simulink model "sampleModel7424_pp_1_1"  (R2018a)
settings: Solver=VariableStepAuto  StartTime=0.0  StopTime=10.0  RelTol=1e-3
undefined symbols (not defined in the file): DiscIntNeverNeededParam
libraries: simulink x211
(part 6 of 7)

== matlab function sampleModel7424_pp_1_1/cfblk142/cfblk19/emi_11 ==
  data: o input; e input
function  fcn(o, e)
o_inv = o^-1;
e_inv = e^-1;

emsg = 'sampleModel7424_pp_1_1/cfblk142/cfblk19/emi_11';
 
if(o == e)
    assert(o_inv == e_inv, [emsg ' ; o_inv~=e_inv']);
    return;
end
 
if(o_inv > 0)
    assert(e_inv < 0, [emsg ' ; e_inv>=0']);
else
    assert(e_inv > 0, [emsg ' ; e_inv<=0']);
end

== matlab function sampleModel7424_pp_1_1/cfblk134/emi_13 ==
  data: o input; e input
function  fcn(o, e)
o_inv = o^-1;
e_inv = e^-1;

emsg = 'sampleModel7424_pp_1_1/cfblk134/emi_13';
 
if(o == e)
    assert(o_inv == e_inv, [emsg ' ; o_inv~=e_inv']);
    return;
end
 
if(o_inv > 0)
    assert(e_inv < 0, [emsg ' ; e_inv>=0']);
else
    assert(e_inv > 0, [emsg ' ; e_inv<=0']);
end

== matlab function sampleModel7424_pp_1_1/cfblk148/emi_15 ==
  data: o input; e input
function  fcn(o, e)
o_inv = o^-1;
e_inv = e^-1;

emsg = 'sampleModel7424_pp_1_1/cfblk148/emi_15';
 
if(o == e)
    assert(o_inv == e_inv, [emsg ' ; o_inv~=e_inv']);
    return;
end
 
if(o_inv > 0)
    assert(e_inv < 0, [emsg ' ; e_inv>=0']);
else
    assert(e_inv > 0, [emsg ' ; e_inv<=0']);
end

== matlab function sampleModel7424_pp_1_1/cfblk127/emi_17 ==
  data: o input; e input
function  fcn(o, e)
o_inv = o^-1;
e_inv = e^-1;

emsg = 'sampleModel7424_pp_1_1/cfblk127/emi_17';
 
if(o == e)
    assert(o_inv == e_inv, [emsg ' ; o_inv~=e_inv']);
    return;
end
 
if(o_inv > 0)
    assert(e_inv < 0, [emsg ' ; e_inv>=0']);
else
    assert(e_inv > 0, [emsg ' ; e_inv<=0']);
end

== matlab function sampleModel7424_pp_1_1/cfblk127/cfblk19/emi_19 ==
  data: o input; e input
function  fcn(o, e)
o_inv = o^-1;
e_inv = e^-1;

emsg = 'sampleModel7424_pp_1_1/cfblk127/cfblk19/emi_19';
 
if(o == e)
    assert(o_inv == e_inv, [emsg ' ; o_inv~=e_inv']);
    return;
end
 
if(o_inv > 0)
    assert(e_inv < 0, [emsg ' ; e_inv>=0']);
else
    assert(e_inv > 0, [emsg ' ; e_inv<=0']);
end

== matlab function sampleModel7424_pp_1_1/emi_21 ==
  data: o input; e input
function  fcn(o, e)
o_inv = o^-1;
e_inv = e^-1;

emsg = 'sampleModel7424_pp_1_1/emi_21';
 
if(o == e)
    assert(o_inv == e_inv, [emsg ' ; o_inv~=e_inv']);
    return;
end
 
if(o_inv > 0)
    assert(e_inv < 0, [emsg ' ; e_inv>=0']);
else
    assert(e_inv > 0, [emsg ' ; e_inv<=0']);
end

== matlab function sampleModel7424_pp_1_1/emi_23 ==
  data: o input; e input
function  fcn(o, e)
o_inv = o^-1;
e_inv = e^-1;

emsg = 'sampleModel7424_pp_1_1/emi_23';
 
if(o == e)
    assert(o_inv == e_inv, [emsg ' ; o_inv~=e_inv']);
    return;
end
 
if(o_inv > 0)
    assert(e_inv < 0, [emsg ' ; e_inv>=0']);
else
    assert(e_inv > 0, [emsg ' ; e_inv<=0']);
end

== matlab function sampleModel7424_pp_1_1/cfblk148/cfblk19/emi_25 ==
  data: o input; e input
function  fcn(o, e)
o_inv = o^-1;
e_inv = e^-1;

emsg = 'sampleModel7424_pp_1_1/cfblk148/cfblk19/emi_25';
 
if(o == e)
    assert(o_inv == e_inv, [emsg ' ; o_inv~=e_inv']);
    return;
end
 
if(o_inv > 0)
    assert(e_inv < 0, [emsg ' ; e_inv>=0']);
else
    assert(e_inv > 0, [emsg ' ; e_inv<=0']);
end

== matlab function sampleModel7424_pp_1_1/cfblk142/emi_27 ==
  data: o input; e input
function  fcn(o, e)
o_inv = o^-1;
e_inv = e^-1;

emsg = 'sampleModel7424_pp_1_1/cfblk142/emi_27';
 
if(o == e)
    assert(o_inv == e_inv, [emsg ' ; o_inv~=e_inv']);
    return;
end
 
if(o_inv > 0)
    assert(e_inv < 0, [emsg ' ; e_inv>=0']);
else
    assert(e_inv > 0, [emsg ' ; e_inv<=0']);
end

== matlab function sampleModel7424_pp_1_1/cfblk148/emi_29 ==
  data: o input; e input
function  fcn(o, e)
o_inv = o^-1;
e_inv = e^-1;

emsg = 'sampleModel7424_pp_1_1/cfblk148/emi_29';
 
if(o == e)
    assert(o_inv == e_inv, [emsg ' ; o_inv~=e_inv']);
    return;
end
 
if(o_inv > 0)
    assert(e_inv < 0, [emsg ' ; e_inv>=0']);
else
    assert(e_inv > 0, [emsg ' ; e_inv<=0']);
end

== matlab function sampleModel7424_pp_1_1/cfblk125/emi_31 ==
  data: o input; e input
function  fcn(o, e)
o_inv = o^-1;
e_inv = e^-1;

emsg = 'sampleModel7424_pp_1_1/cfblk125/emi_31';
 
if(o == e)
    assert(o_inv == e_inv, [emsg ' ; o_inv~=e_inv']);
    return;
end
 
if(o_inv > 0)
    assert(e_inv < 0, [emsg ' ; e_inv>=0']);
else
    assert(e_inv > 0, [emsg ' ; e_inv<=0']);
end

== matlab function sampleModel7424_pp_1_1/cfblk130/cfblk12/emi_33 ==
  data: o input; e input
function  fcn(o, e)
o_inv = o^-1;
e_inv = e^-1;

emsg = 'sampleModel7424_pp_1_1/cfblk130/cfblk12/emi_33';
 
if(o == e)
    assert(o_inv == e_inv, [emsg ' ; o_inv~=e_inv']);
    return;
end
 
if(o_inv > 0)
    assert(e_inv < 0, [emsg ' ; e_inv>=0']);
else
    assert(e_inv > 0, [emsg ' ; e_inv<=0']);
end

== matlab function sampleModel7424_pp_1_1/emi_35 ==
  data: o input; e input
function  fcn(o, e)
o_inv = o^-1;
e_inv = e^-1;

emsg = 'sampleModel7424_pp_1_1/emi_35';
 
if(o == e)
    assert(o_inv == e_inv, [emsg ' ; o_inv~=e_inv']);
    return;
end
 
if(o_inv > 0)
    assert(e_inv < 0, [emsg ' ; e_inv>=0']);
else
    assert(e_inv > 0, [emsg ' ; e_inv<=0']);
end

== matlab function sampleModel7424_pp_1_1/cfblk147/emi_37 ==
  data: o input; e input
function  fcn(o, e)
o_inv = o^-1;
e_inv = e^-1;

emsg = 'sampleModel7424_pp_1_1/cfblk147/emi_37';
 
if(o == e)
    assert(o_inv == e_inv, [emsg ' ; o_inv~=e_inv']);
    return;
end
 
if(o_inv > 0)
    assert(e_inv < 0, [emsg ' ; e_inv>=0']);
else
    assert(e_inv > 0, [emsg ' ; e_inv<=0']);
end

== matlab function sampleModel7424_pp_1_1/cfblk142/emi_39 ==
  data: o input; e input
function  fcn(o, e)
o_inv = o^-1;
e_inv = e^-1;

emsg = 'sampleModel7424_pp_1_1/cfblk142/emi_39';
 
if(o == e)
    assert(o_inv == e_inv, [emsg ' ; o_inv~=e_inv']);
    return;
end
 
if(o_inv > 0)
    assert(e_inv < 0, [emsg ' ; e_inv>=0']);
else
    assert(e_inv > 0, [emsg ' ; e_inv<=0']);
end

== matlab function sampleModel7424_pp_1_1/cfblk136/emi_41 ==
  data: o input; e input
function  fcn(o, e)
o_inv = o^-1;
e_inv = e^-1;

emsg = 'sampleModel7424_pp_1_1/cfblk136/emi_41';
 
if(o == e)
    assert(o_inv == e_inv, [emsg ' ; o_inv~=e_inv']);
    return;
end
 
if(o_inv > 0)
    assert(e_inv < 0, [emsg ' ; e_inv>=0']);
else
    assert(e_inv > 0, [emsg ' ; e_inv<=0']);
end

== matlab function sampleModel7424_pp_1_1/cfblk132/emi_43 ==
  data: o input; e input
function  fcn(o, e)
o_inv = o^-1;
e_inv = e^-1;

emsg = 'sampleModel7424_pp_1_1/cfblk132/emi_43';
 
if(o == e)
    assert(o_inv == e_inv, [emsg ' ; o_inv~=e_inv']);
    return;
end
 
if(o_inv > 0)
    assert(e_inv < 0, [emsg ' ; e_inv>=0']);
else
    assert(e_inv > 0, [emsg ' ; e_inv<=0']);
end

== matlab function sampleModel7424_pp_1_1/cfblk126/cfblk15/emi_45 ==
  data: o input; e input
function  fcn(o, e)
o_inv = o^-1;
e_inv = e^-1;

emsg = 'sampleModel7424_pp_1_1/cfblk126/cfblk15/emi_45';
 
if(o == e)
    assert(o_inv == e_inv, [emsg ' ; o_inv~=e_inv']);
    return;
end
 
if(o_inv > 0)
    assert(e_inv < 0, [emsg ' ; e_inv>=0']);
else
    assert(e_inv > 0, [emsg ' ; e_inv<=0']);
end

== matlab function sampleModel7424_pp_1_1/cfblk134/emi_47 ==
  data: o input; e input
function  fcn(o, e)
o_inv = o^-1;
e_inv = e^-1;

emsg = 'sampleModel7424_pp_1_1/cfblk134/emi_47';
 
if(o == e)
    assert(o_inv == e_inv, [emsg ' ; o_inv~=e_inv']);
    return;
end
 
if(o_inv > 0)
    assert(e_inv < 0, [emsg ' ; e_inv>=0']);
else
    assert(e_inv > 0, [emsg ' ; e_inv<=0']);
end

== matlab function sampleModel7424_pp_1_1/cfblk124/cfblk15/emi_49 ==
  data: o input; e input
function  fcn(o, e)
o_inv = o^-1;
e_inv = e^-1;

emsg = 'sampleModel7424_pp_1_1/cfblk124/cfblk15/emi_49';
 
if(o == e)
    assert(o_inv == e_inv, [emsg ' ; o_inv~=e_inv']);
    return;
end
 
if(o_inv > 0)
    assert(e_inv < 0, [emsg ' ; e_inv>=0']);
else
    assert(e_inv > 0, [emsg ' ; e_inv<=0']);
end

== matlab function sampleModel7424_pp_1_1/cfblk130/emi_51 ==
  data: o input; e input
function  fcn(o, e)
o_inv = o^-1;
e_inv = e^-1;

emsg = 'sampleModel7424_pp_1_1/cfblk130/emi_51';
 
if(o == e)
    assert(o_inv == e_inv, [emsg ' ; o_inv~=e_inv']);
    return;
end
 
if(o_inv > 0)
    assert(e_inv < 0, [emsg ' ; e_inv>=0']);
else
    assert(e_inv > 0, [emsg ' ; e_inv<=0']);
end

== matlab function sampleModel7424_pp_1_1/cfblk125/cfblk12/emi_53 ==
  data: o input; e input
function  fcn(o, e)
o_inv = o^-1;
e_inv = e^-1;

emsg = 'sampleModel7424_pp_1_1/cfblk125/cfblk12/emi_53';
 
if(o == e)
    assert(o_inv == e_inv, [emsg ' ; o_inv~=e_inv']);
    return;
end
 
if(o_inv > 0)
    assert(e_inv < 0, [emsg ' ; e_inv>=0']);
else
    assert(e_inv > 0, [emsg ' ; e_inv<=0']);
end

== matlab function sampleModel7424_pp_1_1/emi_55 ==
  data: o input; e input
function  fcn(o, e)
o_inv = o^-1;
e_inv = e^-1;

emsg = 'sampleModel7424_pp_1_1/emi_55';
 
if(o == e)
    assert(o_inv == e_inv, [emsg ' ; o_inv~=e_inv']);
    return;
end
 
if(o_inv > 0)
    assert(e_inv < 0, [emsg ' ; e_inv>=0']);
else
    assert(e_inv > 0, [emsg ' ; e_inv<=0']);
end

== matlab function sampleModel7424_pp_1_1/cfblk142/cfblk19/emi_57 ==
  data: o input; e input
function  fcn(o, e)
o_inv = o^-1;
e_inv = e^-1;

emsg = 'sampleModel7424_pp_1_1/cfblk142/cfblk19/emi_57';
 
if(o == e)
    assert(o_inv == e_inv, [emsg ' ; o_inv~=e_inv']);
    return;
end
 
if(o_inv > 0)
    assert(e_inv < 0, [emsg ' ; e_inv>=0']);
else
    assert(e_inv > 0, [emsg ' ; e_inv<=0']);
end

== matlab function sampleModel7424_pp_1_1/emi_59 ==
  data: o input; e input
function  fcn(o, e)
o_inv = o^-1;
e_inv = e^-1;

emsg = 'sampleModel7424_pp_1_1/emi_59';
 
if(o == e)
    assert(o_inv == e_inv, [emsg ' ; o_inv~=e_inv']);
    return;
end
 
if(o_inv > 0)
    assert(e_inv < 0, [emsg ' ; e_inv>=0']);
else
    assert(e_inv > 0, [emsg ' ; e_inv<=0']);
end

== matlab function sampleModel7424_pp_1_1/cfblk126/emi_61 ==
  data: o input; e input
function  fcn(o, e)
o_inv = o^-1;
e_inv = e^-1;

emsg = 'sampleModel7424_pp_1_1/cfblk126/emi_61';
 
if(o == e)
    assert(o_inv == e_inv, [emsg ' ; o_inv~=e_inv']);
    return;
end
 
if(o_inv > 0)
    assert(e_inv < 0, [emsg ' ; e_inv>=0']);
else
    assert(e_inv > 0, [emsg ' ; e_inv<=0']);
end

== matlab function sampleModel7424_pp_1_1/cfblk132/emi_63 ==
  data: o input; e input
function  fcn(o, e)
o_inv = o^-1;
e_inv = e^-1;

emsg = 'sampleModel7424_pp_1_1/cfblk132/emi_63';
 
if(o == e)
    assert(o_inv == e_inv, [emsg ' ; o_inv~=e_inv']);
    return;
end
 
if(o_inv > 0)
    assert(e_inv < 0, [emsg ' ; e_inv>=0']);
else
    assert(e_inv > 0, [emsg ' ; e_inv<=0']);
end

== matlab function sampleModel7424_pp_1_1/cfblk130/cfblk12/emi_65 ==
  data: o input; e input
function  fcn(o, e)
o_inv = o^-1;
e_inv = e^-1;

emsg = 'sampleModel7424_pp_1_1/cfblk130/cfblk12/emi_65';
 
if(o == e)
    assert(o_inv == e_inv, [emsg ' ; o_inv~=e_inv']);
    return;
end
 
if(o_inv > 0)
    assert(e_inv < 0, [emsg ' ; e_inv>=0']);
else
    assert(e_inv > 0, [emsg ' ; e_inv<=0']);
end

== matlab function sampleModel7424_pp_1_1/cfblk148/emi_67 ==
  data: o input; e input
function  fcn(o, e)
o_inv = o^-1;
e_inv = e^-1;

emsg = 'sampleModel7424_pp_1_1/cfblk148/emi_67';
 
if(o == e)
    assert(o_inv == e_inv, [emsg ' ; o_inv~=e_inv']);
    return;
end
 
if(o_inv > 0)
    assert(e_inv < 0, [emsg ' ; e_inv>=0']);
else
    assert(e_inv > 0, [emsg ' ; e_inv<=0']);
end

== matlab function sampleModel7424_pp_1_1/cfblk134/cfblk19/emi_69 ==
  data: o input; e input
function  fcn(o, e)
o_inv = o^-1;
e_inv = e^-1;

emsg = 'sampleModel7424_pp_1_1/cfblk134/cfblk19/emi_69';
 
if(o == e)
    assert(o_inv == e_inv, [emsg ' ; o_inv~=e_inv']);
    return;
end
 
if(o_inv > 0)
    assert(e_inv < 0, [emsg ' ; e_inv>=0']);
else
    assert(e_inv > 0, [emsg ' ; e_inv<=0']);
end

== matlab function sampleModel7424_pp_1_1/cfblk124/cfblk15/emi_71 ==
  data: o input; e input
function  fcn(o, e)
o_inv = o^-1;
e_inv = e^-1;

emsg = 'sampleModel7424_pp_1_1/cfblk124/cfblk15/emi_71';
 
if(o == e)
    assert(o_inv == e_inv, [emsg ' ; o_inv~=e_inv']);
    return;
end
 
if(o_inv > 0)
    assert(e_inv < 0, [emsg ' ; e_inv>=0']);
else
    assert(e_inv > 0, [emsg ' ; e_inv<=0']);
end

== matlab function sampleModel7424_pp_1_1/cfblk124/emi_73 ==
  data: o input; e input
function  fcn(o, e)
o_inv = o^-1;
e_inv = e^-1;

emsg = 'sampleModel7424_pp_1_1/cfblk124/emi_73';
 
if(o == e)
    assert(o_inv == e_inv, [emsg ' ; o_inv~=e_inv']);
    return;
end
 
if(o_inv > 0)
    assert(e_inv < 0, [emsg ' ; e_inv>=0']);
else
    assert(e_inv > 0, [emsg ' ; e_inv<=0']);
end

== matlab function sampleModel7424_pp_1_1/cfblk142/cfblk17/emi_75 ==
  data: o input; e input
function  fcn(o, e)
o_inv = o^-1;
e_inv = e^-1;

emsg = 'sampleModel7424_pp_1_1/cfblk142/cfblk17/emi_75';
 
if(o == e)
    assert(o_inv == e_inv, [emsg ' ; o_inv~=e_inv']);
    return;
end
 
if(o_inv > 0)
    assert(e_inv < 0, [emsg ' ; e_inv>=0']);
else
    assert(e_inv > 0, [emsg ' ; e_inv<=0']);
end

== matlab function sampleModel7424_pp_1_1/cfblk134/cfblk19/emi_77 ==
  data: o input; e input
function  fcn(o, e)
o_inv = o^-1;
e_inv = e^-1;

emsg = 'sampleModel7424_pp_1_1/cfblk134/cfblk19/emi_77';
 
if(o == e)
    assert(o_inv == e_inv, [emsg ' ; o_inv~=e_inv']);
    return;
end
 
if(o_inv > 0)
    assert(e_inv < 0, [emsg ' ; e_inv>=0']);
else
    assert(e_inv > 0, [emsg ' ; e_inv<=0']);
end

== matlab function sampleModel7424_pp_1_1/cfblk147/emi_79 ==
  data: o input; e input
function  fcn(o, e)
o_inv = o^-1;
e_inv = e^-1;

emsg = 'sampleModel7424_pp_1_1/cfblk147/emi_79';
 
if(o == e)
    assert(o_inv == e_inv, [emsg ' ; o_inv~=e_inv']);
    return;
end
 
if(o_inv > 0)
    assert(e_inv < 0, [emsg ' ; e_inv>=0']);
else
    assert(e_inv > 0, [emsg ' ; e_inv<=0']);
end

== matlab function sampleModel7424_pp_1_1/cfblk142/cfblk17/emi_81 ==
  data: o input; e input
function  fcn(o, e)
o_inv = o^-1;
e_inv = e^-1;

emsg = 'sampleModel7424_pp_1_1/cfblk142/cfblk17/emi_81';
 
if(o == e)
    assert(o_inv == e_inv, [emsg ' ; o_inv~=e_inv']);
    return;
end
 
if(o_inv > 0)
    assert(e_inv < 0, [emsg ' ; e_inv>=0']);
else
    assert(e_inv > 0, [emsg ' ; e_inv<=0']);
end

== matlab function sampleModel7424_pp_1_1/cfblk126/cfblk15/emi_83 ==
  data: o input; e input
function  fcn(o, e)
o_inv = o^-1;
e_inv = e^-1;

emsg = 'sampleModel7424_pp_1_1/cfblk126/cfblk15/emi_83';
 
if(o == e)
    assert(o_inv == e_inv, [emsg ' ; o_inv~=e_inv']);
    return;
end
 
if(o_inv > 0)
    assert(e_inv < 0, [emsg ' ; e_inv>=0']);
else
    assert(e_inv > 0, [emsg ' ; e_inv<=0']);
end

== matlab function sampleModel7424_pp_1_1/cfblk136/emi_85 ==
  data: o input; e input
function  fcn(o, e)
o_inv = o^-1;
e_inv = e^-1;

emsg = 'sampleModel7424_pp_1_1/cfblk136/emi_85';
 
if(o == e)
    assert(o_inv == e_inv, [emsg ' ; o_inv~=e_inv']);
    return;
end
 
if(o_inv > 0)
    assert(e_inv < 0, [emsg ' ; e_inv>=0']);
else
    assert(e_inv > 0, [emsg ' ; e_inv<=0']);
end

== matlab function sampleModel7424_pp_1_1/cfblk142/cfblk19/emi_87 ==
  data: o input; e input
function  fcn(o, e)
o_inv = o^-1;
e_inv = e^-1;

emsg = 'sampleModel7424_pp_1_1/cfblk142/cfblk19/emi_87';
 
if(o == e)
    assert(o_inv == e_inv, [emsg ' ; o_inv~=e_inv']);
    return;
end
 
if(o_inv > 0)
    assert(e_inv < 0, [emsg ' ; e_inv>=0']);
else
    assert(e_inv > 0, [emsg ' ; e_inv<=0']);
end

== matlab function sampleModel7424_pp_1_1/cfblk133/emi_89 ==
  data: o input; e input
function  fcn(o, e)
o_inv = o^-1;
e_inv = e^-1;

emsg = 'sampleModel7424_pp_1_1/cfblk133/emi_89';
 
if(o == e)
    assert(o_inv == e_inv, [emsg ' ; o_inv~=e_inv']);
    return;
end
 
if(o_inv > 0)
    assert(e_inv < 0, [emsg ' ; e_inv>=0']);
else
    assert(e_inv > 0, [emsg ' ; e_inv<=0']);
end

== matlab function sampleModel7424_pp_1_1/cfblk130/cfblk12/emi_91 ==
  data: o input; e input
function  fcn(o, e)
o_inv = o^-1;
e_inv = e^-1;

emsg = 'sampleModel7424_pp_1_1/cfblk130/cfblk12/emi_91';
 
if(o == e)
    assert(o_inv == e_inv, [emsg ' ; o_inv~=e_inv']);
    return;
end
 
if(o_inv > 0)
    assert(e_inv < 0, [emsg ' ; e_inv>=0']);
else
    assert(e_inv > 0, [emsg ' ; e_inv<=0']);
end

== matlab function sampleModel7424_pp_1_1/emi_93 ==
  data: o input; e input
function  fcn(o, e)
o_inv = o^-1;
e_inv = e^-1;

emsg = 'sampleModel7424_pp_1_1/emi_93';
 
if(o == e)
    assert(o_inv == e_inv, [emsg ' ; o_inv~=e_inv']);
    return;
end
 
if(o_inv > 0)
    assert(e_inv < 0, [emsg ' ; e_inv>=0']);
else
    assert(e_inv > 0, [emsg ' ; e_inv<=0']);
end

== matlab function sampleModel7424_pp_1_1/cfblk126/emi_95 ==
  data: o input; e input
function  fcn(o, e)
o_inv = o^-1;
e_inv = e^-1;

emsg = 'sampleModel7424_pp_1_1/cfblk126/emi_95';
 
if(o == e)
    assert(o_inv == e_inv, [emsg ' ; o_inv~=e_inv']);
    return;
end
 
if(o_inv > 0)
    assert(e_inv < 0, [emsg ' ; e_inv>=0']);
else
    assert(e_inv > 0, [emsg ' ; e_inv<=0']);
end

== matlab function sampleModel7424_pp_1_1/emi_97 ==
  data: o input; e input
function  fcn(o, e)
o_inv = o^-1;
e_inv = e^-1;

emsg = 'sampleModel7424_pp_1_1/emi_97';
 
if(o == e)
    assert(o_inv == e_inv, [emsg ' ; o_inv~=e_inv']);
    return;
end
 
if(o_inv > 0)
    assert(e_inv < 0, [emsg ' ; e_inv>=0']);
else
    assert(e_inv > 0, [emsg ' ; e_inv<=0']);
end

== matlab function sampleModel7424_pp_1_1/cfblk125/cfblk12/emi_99 ==
  data: o input; e input
function  fcn(o, e)
o_inv = o^-1;
e_inv = e^-1;

emsg = 'sampleModel7424_pp_1_1/cfblk125/cfblk12/emi_99';
 
if(o == e)
    assert(o_inv == e_inv, [emsg ' ; o_inv~=e_inv']);
    return;
end
 
if(o_inv > 0)
    assert(e_inv < 0, [emsg ' ; e_inv>=0']);
else
    assert(e_inv > 0, [emsg ' ; e_inv<=0']);
end

== matlab function sampleModel7424_pp_1_1/cfblk124/emi_101 ==
  data: o input; e input
function  fcn(o, e)
o_inv = o^-1;
e_inv = e^-1;

emsg = 'sampleModel7424_pp_1_1/cfblk124/emi_101';
 
if(o == e)
    assert(o_inv == e_inv, [emsg ' ; o_inv~=e_inv']);
    return;
end
 
if(o_inv > 0)
    assert(e_inv < 0, [emsg ' ; e_inv>=0']);
else
    assert(e_inv > 0, [emsg ' ; e_inv<=0']);
end

== matlab function sampleModel7424_pp_1_1/cfblk124/emi_103 ==
  data: o input; e input
function  fcn(o, e)
o_inv = o^-1;
e_inv = e^-1;

emsg = 'sampleModel7424_pp_1_1/cfblk124/emi_103';
 
if(o == e)
    assert(o_inv == e_inv, [emsg ' ; o_inv~=e_inv']);
    return;
end
 
if(o_inv > 0)
    assert(e_inv < 0, [emsg ' ; e_inv>=0']);
else
    assert(e_inv > 0, [emsg ' ; e_inv<=0']);
end

== matlab function sampleModel7424_pp_1_1/emi_105 ==
  data: o input; e input
function  fcn(o, e)
o_inv = o^-1;
e_inv = e^-1;

emsg = 'sampleModel7424_pp_1_1/emi_105';
 
if(o == e)
    assert(o_inv == e_inv, [emsg ' ; o_inv~=e_inv']);
    return;
end
 
if(o_inv > 0)
    assert(e_inv < 0, [emsg ' ; e_inv>=0']);
else
    assert(e_inv > 0, [emsg ' ; e_inv<=0']);
end

== matlab function sampleModel7424_pp_1_1/cfblk148/cfblk19/emi_107 ==
  data: o input; e input
function  fcn(o, e)
o_inv = o^-1;
e_inv = e^-1;

emsg = 'sampleModel7424_pp_1_1/cfblk148/cfblk19/emi_107';
 
if(o == e)
    assert(o_inv == e_inv, [emsg ' ; o_inv~=e_inv']);
    return;
end
 
if(o_inv > 0)
    assert(e_inv < 0, [emsg ' ; e_inv>=0']);
else
    assert(e_inv > 0, [emsg ' ; e_inv<=0']);
end

== matlab function sampleModel7424_pp_1_1/emi_109 ==
  data: o input; e input
function  fcn(o, e)
o_inv = o^-1;
e_inv = e^-1;

emsg = 'sampleModel7424_pp_1_1/emi_109';
 
if(o == e)
    assert(o_inv == e_inv, [emsg ' ; o_inv~=e_inv']);
    return;
end
 
if(o_inv > 0)
    assert(e_inv < 0, [emsg ' ; e_inv>=0']);
else
    assert(e_inv > 0, [emsg ' ; e_inv<=0']);
end

== matlab function sampleModel7424_pp_1_1/cfblk148/emi_111 ==
  data: o input; e input
function  fcn(o, e)
o_inv = o^-1;
e_inv = e^-1;

emsg = 'sampleModel7424_pp_1_1/cfblk148/emi_111';
 
if(o == e)
    assert(o_inv == e_inv, [emsg ' ; o_inv~=e_inv']);
    return;
end
 
if(o_inv > 0)
    assert(e_inv < 0, [emsg ' ; e_inv>=0']);
else
    assert(e_inv > 0, [emsg ' ; e_inv<=0']);
end

== matlab function sampleModel7424_pp_1_1/cfblk124/cfblk17/emi_113 ==
  data: o input; e input
function  fcn(o, e)
o_inv = o^-1;
e_inv = e^-1;

emsg = 'sampleModel7424_pp_1_1/cfblk124/cfblk17/emi_113';
 
if(o == e)
    assert(o_inv == e_inv, [emsg ' ; o_inv~=e_inv']);
    return;
end
 
if(o_inv > 0)
    assert(e_inv < 0, [emsg ' ; e_inv>=0']);
else
    assert(e_inv > 0, [emsg ' ; e_inv<=0']);
end

== matlab function sampleModel7424_pp_1_1/cfblk142/emi_115 ==
  data: o input; e input
function  fcn(o, e)
o_inv = o^-1;
e_inv = e^-1;

emsg = 'sampleModel7424_pp_1_1/cfblk142/emi_115';
 
if(o == e)
    assert(o_inv == e_inv, [emsg ' ; o_inv~=e_inv']);
    return;
end
 
if(o_inv > 0)
    assert(e_inv < 0, [emsg ' ; e_inv>=0']);
else
    assert(e_inv > 0, [emsg ' ; e_inv<=0']);
end

== matlab function sampleModel7424_pp_1_1/cfblk133/emi_117 ==
  data: o input; e input
function  fcn(o, e)
o_inv = o^-1;
e_inv = e^-1;

emsg = 'sampleModel7424_pp_1_1/cfblk133/emi_117';
 
if(o == e)
    assert(o_inv == e_inv, [emsg ' ; o_inv~=e_inv']);
    return;
end
 
if(o_inv > 0)
    assert(e_inv < 0, [emsg ' ; e_inv>=0']);
else
    assert(e_inv > 0, [emsg ' ; e_inv<=0']);
end

== matlab function sampleModel7424_pp_1_1/cfblk140/emi_119 ==
  data: o input; e input
function  fcn(o, e)
o_inv = o^-1;
e_inv = e^-1;

emsg = 'sampleModel7424_pp_1_1/cfblk140/emi_119';
 
if(o == e)
    assert(o_inv == e_inv, [emsg ' ; o_inv~=e_inv']);
    return;
end
 
if(o_inv > 0)
    assert(e_inv < 0, [emsg ' ; e_inv>=0']);
else
    assert(e_inv > 0, [emsg ' ; e_inv<=0']);
end

== matlab function sampleModel7424_pp_1_1/cfblk126/cfblk15/emi_121 ==
  data: o input; e input
function  fcn(o, e)
o_inv = o^-1;
e_inv = e^-1;

emsg = 'sampleModel7424_pp_1_1/cfblk126/cfblk15/emi_121';
 
if(o == e)
    assert(o_inv == e_inv, [emsg ' ; o_inv~=e_inv']);
    return;
end
 
if(o_inv > 0)
    assert(e_inv < 0, [emsg ' ; e_inv>=0']);
else
    assert(e_inv > 0, [emsg ' ; e_inv<=0']);
end

== matlab function sampleModel7424_pp_1_1/cfblk125/cfblk12/emi_123 ==
  data: o input; e input
function  fcn(o, e)
o_inv = o^-1;
e_inv = e^-1;

emsg = 'sampleModel7424_pp_1_1/cfblk125/cfblk12/emi_123';
 
if(o == e)
    assert(o_inv == e_inv, [emsg ' ; o_inv~=e_inv']);
    return;
end
 
if(o_inv > 0)
    assert(e_inv < 0, [emsg ' ; e_inv>=0']);
else
    assert(e_inv > 0, [emsg ' ; e_inv<=0']);
end

== matlab function sampleModel7424_pp_1_1/emi_125 ==
  data: o input; e input
function  fcn(o, e)
o_inv = o^-1;
e_inv = e^-1;

emsg = 'sampleModel7424_pp_1_1/emi_125';
 
if(o == e)
    assert(o_inv == e_inv, [emsg ' ; o_inv~=e_inv']);
    return;
end
 
if(o_inv > 0)
    assert(e_inv < 0, [emsg ' ; e_inv>=0']);
else
    assert(e_inv > 0, [emsg ' ; e_inv<=0']);
end

== matlab function sampleModel7424_pp_1_1/cfblk127/emi_127 ==
  data: o input; e input
function  fcn(o, e)
o_inv = o^-1;
e_inv = e^-1;

emsg = 'sampleModel7424_pp_1_1/cfblk127/emi_127';
 
if(o == e)
    assert(o_inv == e_inv, [emsg ' ; o_inv~=e_inv']);
    return;
end
 
if(o_inv > 0)
    assert(e_inv < 0, [emsg ' ; e_inv>=0']);
else
    assert(e_inv > 0, [emsg ' ; e_inv<=0']);
end

== matlab function sampleModel7424_pp_1_1/cfblk148/cfblk19/emi_129 ==
  data: o input; e input
function  fcn(o, e)
o_inv = o^-1;
e_inv = e^-1;

emsg = 'sampleModel7424_pp_1_1/cfblk148/cfblk19/emi_129';
 
if(o == e)
    assert(o_inv == e_inv, [emsg ' ; o_inv~=e_inv']);
    return;
end
 
if(o_inv > 0)
    assert(e_inv < 0, [emsg ' ; e_inv>=0']);
else
    assert(e_inv > 0, [emsg ' ; e_inv<=0']);
end

== matlab function sampleModel7424_pp_1_1/emi_131 ==
  data: o input; e input
function  fcn(o, e)
o_inv = o^-1;
e_inv = e^-1;

emsg = 'sampleModel7424_pp_1_1/emi_131';
 
if(o == e)
    assert(o_inv == e_inv, [emsg ' ; o_inv~=e_inv']);
    return;
end
 
if(o_inv > 0)
    assert(e_inv < 0, [emsg ' ; e_inv>=0']);
else
    assert(e_inv > 0, [emsg ' ; e_inv<=0']);
end

== matlab function sampleModel7424_pp_1_1/cfblk148/emi_133 ==
  data: o input; e input
function  fcn(o, e)
o_inv = o^-1;
e_inv = e^-1;

emsg = 'sampleModel7424_pp_1_1/cfblk148/emi_133';
 
if(o == e)
    assert(o_inv == e_inv, [emsg ' ; o_inv~=e_inv']);
    return;
end
 
if(o_inv > 0)
    assert(e_inv < 0, [emsg ' ; e_inv>=0']);
else
    assert(e_inv > 0, [emsg ' ; e_inv<=0']);
end

== matlab function sampleModel7424_pp_1_1/cfblk132/emi_135 ==
  data: o input; e input
function  fcn(o, e)
o_inv = o^-1;
e_inv = e^-1;

emsg = 'sampleModel7424_pp_1_1/cfblk132/emi_135';
 
if(o == e)
    assert(o_inv == e_inv, [emsg ' ; o_inv~=e_inv']);
    return;
end
 
if(o_inv > 0)
    assert(e_inv < 0, [emsg ' ; e_inv>=0']);
else
    assert(e_inv > 0, [emsg ' ; e_inv<=0']);
end

== matlab function sampleModel7424_pp_1_1/cfblk148/cfblk19/emi_137 ==
  data: o input; e input
function  fcn(o, e)
o_inv = o^-1;
e_inv = e^-1;

emsg = 'sampleModel7424_pp_1_1/cfblk148/cfblk19/emi_137';
 
if(o == e)
    assert(o_inv == e_inv, [emsg ' ; o_inv~=e_inv']);
    return;
end
 
if(o_inv > 0)
    assert(e_inv < 0, [emsg ' ; e_inv>=0']);
else
    assert(e_inv > 0, [emsg ' ; e_inv<=0']);
end

== matlab function sampleModel7424_pp_1_1/cfblk132/emi_139 ==
  data: o input; e input
function  fcn(o, e)
o_inv = o^-1;
e_inv = e^-1;

emsg = 'sampleModel7424_pp_1_1/cfblk132/emi_139';
 
if(o == e)
    assert(o_inv == e_inv, [emsg ' ; o_inv~=e_inv']);
    return;
end
 
if(o_inv > 0)
    assert(e_inv < 0, [emsg ' ; e_inv>=0']);
else
    assert(e_inv > 0, [emsg ' ; e_inv<=0']);
end

== matlab function sampleModel7424_pp_1_1/cfblk148/cfblk19/emi_141 ==
  data: o input; e input
function  fcn(o, e)
o_inv = o^-1;
e_inv = e^-1;

emsg = 'sampleModel7424_pp_1_1/cfblk148/cfblk19/emi_141';
 
if(o == e)
    assert(o_inv == e_inv, [emsg ' ; o_inv~=e_inv']);
    return;
end
 
if(o_inv > 0)
    assert(e_inv < 0, [emsg ' ; e_inv>=0']);
else
    assert(e_inv > 0, [emsg ' ; e_inv<=0']);
end

== matlab function sampleModel7424_pp_1_1/cfblk141/emi_143 ==
  data: o input; e input
function  fcn(o, e)
o_inv = o^-1;
e_inv = e^-1;

emsg = 'sampleModel7424_pp_1_1/cfblk141/emi_143';
 
if(o == e)
    assert(o_inv == e_inv, [emsg ' ; o_inv~=e_inv']);
    return;
end
 
if(o_inv > 0)
    assert(e_inv < 0, [emsg ' ; e_inv>=0']);
else
    assert(e_inv > 0, [emsg ' ; e_inv<=0']);
end

== matlab function sampleModel7424_pp_1_1/cfblk138/emi_145 ==
  data: o input; e input
function  fcn(o, e)
o_inv = o^-1;
e_inv = e^-1;

emsg = 'sampleModel7424_pp_1_1/cfblk138/emi_145';
 
if(o == e)
    assert(o_inv == e_inv, [emsg ' ; o_inv~=e_inv']);
    return;
end
 
if(o_inv > 0)
    assert(e_inv < 0, [emsg ' ; e_inv>=0']);
else
    assert(e_inv > 0, [emsg ' ; e_inv<=0']);
end

== matlab function sampleModel7424_pp_1_1/cfblk148/cfblk19/emi_147 ==
  data: o input; e input
function  fcn(o, e)
o_inv = o^-1;
e_inv = e^-1;

emsg = 'sampleModel7424_pp_1_1/cfblk148/cfblk19/emi_147';
 
if(o == e)
    assert(o_inv == e_inv, [emsg ' ; o_inv~=e_inv']);
    return;
end
 
if(o_inv > 0)
    assert(e_inv < 0, [emsg ' ; e_inv>=0']);
else
    assert(e_inv > 0, [emsg ' ; e_inv<=0']);
end

== matlab function sampleModel7424_pp_1_1/cfblk134/cfblk19/emi_149 ==
  data: o input; e input
function  fcn(o, e)
o_inv = o^-1;
e_inv = e^-1;

emsg = 'sampleModel7424_pp_1_1/cfblk134/cfblk19/emi_149';
 
if(o == e)
    assert(o_inv == e_inv, [emsg ' ; o_inv~=e_inv']);
    return;
end
 
if(o_inv > 0)
    assert(e_inv < 0, [emsg ' ; e_inv>=0']);
else
    assert(e_inv > 0, [emsg ' ; e_inv<=0']);
end

== matlab function sampleModel7424_pp_1_1/cfblk130/cfblk12/emi_151 ==
  data: o input; e input
function  fcn(o, e)
o_inv = o^-1;
e_inv = e^-1;

emsg = 'sampleModel7424_pp_1_1/cfblk130/cfblk12/emi_151';
 
if(o == e)
    assert(o_inv == e_inv, [emsg ' ; o_inv~=e_inv']);
    return;
end
 
if(o_inv > 0)
    assert(e_inv < 0, [emsg ' ; e_inv>=0']);
else
    assert(e_inv > 0, [emsg ' ; e_inv<=0']);
end

== matlab function sampleModel7424_pp_1_1/cfblk124/cfblk15/emi_153 ==
  data: o input; e input
function  fcn(o, e)
o_inv = o^-1;
e_inv = e^-1;

emsg = 'sampleModel7424_pp_1_1/cfblk124/cfblk15/emi_153';
 
if(o == e)
    assert(o_inv == e_inv, [emsg ' ; o_inv~=e_inv']);
    return;
end
 
if(o_inv > 0)
    assert(e_inv < 0, [emsg ' ; e_inv>=0']);
else
    assert(e_inv > 0, [emsg ' ; e_inv<=0']);
end

== matlab function sampleModel7424_pp_1_1/cfblk124/emi_155 ==
  data: o input; e input
function  fcn(o, e)
o_inv = o^-1;
e_inv = e^-1;

emsg = 'sampleModel7424_pp_1_1/cfblk124/emi_155';
 
if(o == e)
    assert(o_inv == e_inv, [emsg ' ; o_inv~=e_inv']);
    return;
end
 
if(o_inv > 0)
    assert(e_inv < 0, [emsg ' ; e_inv>=0']);
else
    assert(e_inv > 0, [emsg ' ; e_inv<=0']);
end

== matlab function sampleModel7424_pp_1_1/cfblk125/cfblk12/emi_157 ==
  data: o input; e input
function  fcn(o, e)
o_inv = o^-1;
e_inv = e^-1;

emsg = 'sampleModel7424_pp_1_1/cfblk125/cfblk12/emi_157';
 
if(o == e)
    assert(o_inv == e_inv, [emsg ' ; o_inv~=e_inv']);
    return;
end
 
if(o_inv > 0)
    assert(e_inv < 0, [emsg ' ; e_inv>=0']);
else
    assert(e_inv > 0, [emsg ' ; e_inv<=0']);
end

== matlab function sampleModel7424_pp_1_1/cfblk147/emi_159 ==
  data: o input; e input
function  fcn(o, e)
o_inv = o^-1;
e_inv = e^-1;

emsg = 'sampleModel7424_pp_1_1/cfblk147/emi_159';
 
if(o == e)
    assert(o_inv == e_inv, [emsg ' ; o_inv~=e_inv']);
    return;
end
 
if(o_inv > 0)
    assert(e_inv < 0, [emsg ' ; e_inv>=0']);
else
    assert(e_inv > 0, [emsg ' ; e_inv<=0']);
end

== matlab function sampleModel7424_pp_1_1/emi_161 ==
  data: o input; e input
function  fcn(o, e)
o_inv = o^-1;
e_inv = e^-1;

emsg = 'sampleModel7424_pp_1_1/emi_161';
 
if(o == e)
    assert(o_inv == e_inv, [emsg ' ; o_inv~=e_inv']);
    return;
end
 
if(o_inv > 0)
    assert(e_inv < 0, [emsg ' ; e_inv>=0']);
else
    assert(e_inv > 0, [emsg ' ; e_inv<=0']);
end

== matlab function sampleModel7424_pp_1_1/cfblk148/cfblk19/emi_163 ==
  data: o input; e input
function  fcn(o, e)
o_inv = o^-1;
e_inv = e^-1;

emsg = 'sampleModel7424_pp_1_1/cfblk148/cfblk19/emi_163';
 
if(o == e)
    assert(o_inv == e_inv, [emsg ' ; o_inv~=e_inv']);
    return;
end
 
if(o_inv > 0)
    assert(e_inv < 0, [emsg ' ; e_inv>=0']);
else
    assert(e_inv > 0, [emsg ' ; e_inv<=0']);
end

== matlab function sampleModel7424_pp_1_1/cfblk130/cfblk12/emi_165 ==
  data: o input; e input
function  fcn(o, e)
o_inv = o^-1;
e_inv = e^-1;

emsg = 'sampleModel7424_pp_1_1/cfblk130/cfblk12/emi_165';
 
if(o == e)
    assert(o_inv == e_inv, [emsg ' ; o_inv~=e_inv']);
    return;
end
 
if(o_inv > 0)
    assert(e_inv < 0, [emsg ' ; e_inv>=0']);
else
    assert(e_inv > 0, [emsg ' ; e_inv<=0']);
end

== matlab function sampleModel7424_pp_1_1/cfblk130/cfblk12/emi_167 ==
  data: o input; e input
function  fcn(o, e)
o_inv = o^-1;
e_inv = e^-1;

emsg = 'sampleModel7424_pp_1_1/cfblk130/cfblk12/emi_167';
 
if(o == e)
    assert(o_inv == e_inv, [emsg ' ; o_inv~=e_inv']);
    return;
end
 
if(o_inv > 0)
    assert(e_inv < 0, [emsg ' ; e_inv>=0']);
else
    assert(e_inv > 0, [emsg ' ; e_inv<=0']);
end

== matlab function sampleModel7424_pp_1_1/emi_169 ==
  data: o input; e input
function  fcn(o, e)
o_inv = o^-1;
e_inv = e^-1;

emsg = 'sampleModel7424_pp_1_1/emi_169';
 
if(o == e)
    assert(o_inv == e_inv, [emsg ' ; o_inv~=e_inv']);
    return;
end
 
if(o_inv > 0)
    assert(e_inv < 0, [emsg ' ; e_inv>=0']);
else
    assert(e_inv > 0, [emsg ' ; e_inv<=0']);
end

== matlab function sampleModel7424_pp_1_1/cfblk142/cfblk19/emi_171 ==
  data: o input; e input
function  fcn(o, e)
o_inv = o^-1;
e_inv = e^-1;

emsg = 'sampleModel7424_pp_1_1/cfblk142/cfblk19/emi_171';
 
if(o == e)
    assert(o_inv == e_inv, [emsg ' ; o_inv~=e_inv']);
    return;
end
 
if(o_inv > 0)
    assert(e_inv < 0, [emsg ' ; e_inv>=0']);
else
    assert(e_inv > 0, [emsg ' ; e_inv<=0']);
end

== matlab function sampleModel7424_pp_1_1/cfblk134/emi_173 ==
  data: o input; e input
function  fcn(o, e)
o_inv = o^-1;
e_inv = e^-1;

emsg = 'sampleModel7424_pp_1_1/cfblk134/emi_173';
 
if(o == e)
    assert(o_inv == e_inv, [emsg ' ; o_inv~=e_inv']);
    return;
end
 
if(o_inv > 0)
    assert(e_inv < 0, [emsg ' ; e_inv>=0']);
else
    assert(e_inv > 0, [emsg ' ; e_inv<=0']);
end

== matlab function sampleModel7424_pp_1_1/cfblk138/emi_175 ==
  data: o input; e input
function  fcn(o, e)
o_inv = o^-1;
e_inv = e^-1;

emsg = 'sampleModel7424_pp_1_1/cfblk138/emi_175';
 
if(o == e)
    assert(o_inv == e_inv, [emsg ' ; o_inv~=e_inv']);
    return;
end
 
if(o_inv > 0)
    assert(e_inv < 0, [emsg ' ; e_inv>=0']);
else
    assert(e_inv > 0, [emsg ' ; e_inv<=0']);
end

== matlab function sampleModel7424_pp_1_1/emi_177 ==
  data: o input; e input
function  fcn(o, e)
o_inv = o^-1;
e_inv = e^-1;

emsg = 'sampleModel7424_pp_1_1/emi_177';
 
if(o == e)
    assert(o_inv == e_inv, [emsg ' ; o_inv~=e_inv']);
    return;
end
 
if(o_inv > 0)
    assert(e_inv < 0, [emsg ' ; e_inv>=0']);
else
    assert(e_inv > 0, [emsg ' ; e_inv<=0']);
end

== matlab function sampleModel7424_pp_1_1/cfblk148/emi_179 ==
  data: o input; e input
function  fcn(o, e)
o_inv = o^-1;
e_inv = e^-1;

emsg = 'sampleModel7424_pp_1_1/cfblk148/emi_179';
 
if(o == e)
    assert(o_inv == e_inv, [emsg ' ; o_inv~=e_inv']);
    return;
end
 
if(o_inv > 0)
    assert(e_inv < 0, [emsg ' ; e_inv>=0']);
else
    assert(e_inv > 0, [emsg ' ; e_inv<=0']);
end

== matlab function sampleModel7424_pp_1_1/cfblk125/cfblk12/emi_181 ==
  data: o input; e input
function  fcn(o, e)
o_inv = o^-1;
e_inv = e^-1;

emsg = 'sampleModel7424_pp_1_1/cfblk125/cfblk12/emi_181';
 
if(o == e)
    assert(o_inv == e_inv, [emsg ' ; o_inv~=e_inv']);
    return;
end
 
if(o_inv > 0)
    assert(e_inv < 0, [emsg ' ; e_inv>=0']);
else
    assert(e_inv > 0, [emsg ' ; e_inv<=0']);
end

== matlab function sampleModel7424_pp_1_1/cfblk136/emi_183 ==
  data: o input; e input
function  fcn(o, e)
o_inv = o^-1;
e_inv = e^-1;

emsg = 'sampleModel7424_pp_1_1/cfblk136/emi_183';
 
if(o == e)
    assert(o_inv == e_inv, [emsg ' ; o_inv~=e_inv']);
    return;
end
 
if(o_inv > 0)
    assert(e_inv < 0, [emsg ' ; e_inv>=0']);
else
    assert(e_inv > 0, [emsg ' ; e_inv<=0']);
end

== matlab function sampleModel7424_pp_1_1/cfblk134/emi_185 ==
  data: o input; e input
function  fcn(o, e)
o_inv = o^-1;
e_inv = e^-1;

emsg = 'sampleModel7424_pp_1_1/cfblk134/emi_185';
 
if(o == e)
    assert(o_inv == e_inv, [emsg ' ; o_inv~=e_inv']);
    return;
end
 
if(o_inv > 0)
    assert(e_inv < 0, [emsg ' ; e_inv>=0']);
else
    assert(e_inv > 0, [emsg ' ; e_inv<=0']);
end

== matlab function sampleModel7424_pp_1_1/cfblk142/emi_187 ==
  data: o input; e input
function  fcn(o, e)
o_inv = o^-1;
e_inv = e^-1;

emsg = 'sampleModel7424_pp_1_1/cfblk142/emi_187';
 
if(o == e)
    assert(o_inv == e_inv, [emsg ' ; o_inv~=e_inv']);
    return;
end
 
if(o_inv > 0)
    assert(e_inv < 0, [emsg ' ; e_inv>=0']);
else
    assert(e_inv > 0, [emsg ' ; e_inv<=0']);
end

== matlab function sampleModel7424_pp_1_1/cfblk130/cfblk12/emi_189 ==
  data: o input; e input
function  fcn(o, e)
o_inv = o^-1;
e_inv = e^-1;

emsg = 'sampleModel7424_pp_1_1/cfblk130/cfblk12/emi_189';
 
if(o == e)
    assert(o_inv == e_inv, [emsg ' ; o_inv~=e_inv']);
    return;
end
 
if(o_inv > 0)
    assert(e_inv < 0, [emsg ' ; e_inv>=0']);
else
    assert(e_inv > 0, [emsg ' ; e_inv<=0']);
end

== matlab function sampleModel7424_pp_1_1/emi_191 ==
  data: o input; e input
function  fcn(o, e)
o_inv = o^-1;
e_inv = e^-1;

emsg = 'sampleModel7424_pp_1_1/emi_191';
 
if(o == e)
    assert(o_inv == e_inv, [emsg ' ; o_inv~=e_inv']);
    return;
end
 
if(o_inv > 0)
    assert(e_inv < 0, [emsg ' ; e_inv>=0']);
else
    assert(e_inv > 0, [emsg ' ; e_inv<=0']);
end

== matlab function sampleModel7424_pp_1_1/emi_193 ==
  data: o input; e input
function  fcn(o, e)
o_inv = o^-1;
e_inv = e^-1;

emsg = 'sampleModel7424_pp_1_1/emi_193';
 
if(o == e)
    assert(o_inv == e_inv, [emsg ' ; o_inv~=e_inv']);
    return;
end
 
if(o_inv > 0)
    assert(e_inv < 0, [emsg ' ; e_inv>=0']);
else
    assert(e_inv > 0, [emsg ' ; e_inv<=0']);
end

== matlab function sampleModel7424_pp_1_1/emi_195 ==
  data: o input; e input
function  fcn(o, e)
o_inv = o^-1;
e_inv = e^-1;

emsg = 'sampleModel7424_pp_1_1/emi_195';
 
if(o == e)
    assert(o_inv == e_inv, [emsg ' ; o_inv~=e_inv']);
    return;
end
 
if(o_inv > 0)
    assert(e_inv < 0, [emsg ' ; e_inv>=0']);
else
    assert(e_inv > 0, [emsg ' ; e_inv<=0']);
end

== matlab function sampleModel7424_pp_1_1/cfblk144/emi_197 ==
  data: o input; e input
function  fcn(o, e)
o_inv = o^-1;
e_inv = e^-1;

emsg = 'sampleModel7424_pp_1_1/cfblk144/emi_197';
 
if(o == e)
    assert(o_inv == e_inv, [emsg ' ; o_inv~=e_inv']);
    return;
end
 
if(o_inv > 0)
    assert(e_inv < 0, [emsg ' ; e_inv>=0']);
else
    assert(e_inv > 0, [emsg ' ; e_inv<=0']);
end

== matlab function sampleModel7424_pp_1_1/cfblk132/emi_199 ==
  data: o input; e input
function  fcn(o, e)
o_inv = o^-1;
e_inv = e^-1;

emsg = 'sampleModel7424_pp_1_1/cfblk132/emi_199';
 
if(o == e)
    assert(o_inv == e_inv, [emsg ' ; o_inv~=e_inv']);
    return;
end
 
if(o_inv > 0)
    assert(e_inv < 0, [emsg ' ; e_inv>=0']);
else
    assert(e_inv > 0, [emsg ' ; e_inv<=0']);
end

== matlab function sampleModel7424_pp_1_1/cfblk148/cfblk19/emi_201 ==
  data: o input; e input
function  fcn(o, e)
o_inv = o^-1;
e_inv = e^-1;

emsg = 'sampleModel7424_pp_1_1/cfblk148/cfblk19/emi_201';
 
if(o == e)
    assert(o_inv == e_inv, [emsg ' ; o_inv~=e_inv']);
    return;
end
 
if(o_inv > 0)
    assert(e_inv < 0, [emsg ' ; e_inv>=0']);
else
    assert(e_inv > 0, [emsg ' ; e_inv<=0']);
end

== matlab function sampleModel7424_pp_1_1/cfblk126/cfblk15/emi_203 ==
  data: o input; e input
function  fcn(o, e)
o_inv = o^-1;
e_inv = e^-1;

emsg = 'sampleModel7424_pp_1_1/cfblk126/cfblk15/emi_203';
 
if(o == e)
    assert(o_inv == e_inv, [emsg ' ; o_inv~=e_inv']);
    return;
end
 
if(o_inv > 0)
    assert(e_inv < 0, [emsg ' ; e_inv>=0']);
else
    assert(e_inv > 0, [emsg ' ; e_inv<=0']);
end

== matlab function sampleModel7424_pp_1_1/emi_205 ==
  data: o input; e input
function  fcn(o, e)
o_inv = o^-1;
e_inv = e^-1;

emsg = 'sampleModel7424_pp_1_1/emi_205';
 
if(o == e)
    assert(o_inv == e_inv, [emsg ' ; o_inv~=e_inv']);
    return;
end
 
if(o_inv > 0)
    assert(e_inv < 0, [emsg ' ; e_inv>=0']);
else
    assert(e_inv > 0, [emsg ' ; e_inv<=0']);
end

== matlab function sampleModel7424_pp_1_1/cfblk124/emi_207 ==
  data: o input; e input
function  fcn(o, e)
o_inv = o^-1;
e_inv = e^-1;

emsg = 'sampleModel7424_pp_1_1/cfblk124/emi_207';
 
if(o == e)
    assert(o_inv == e_inv, [emsg ' ; o_inv~=e_inv']);
    return;
end
 
if(o_inv > 0)
    assert(e_inv < 0, [emsg ' ; e_inv>=0']);
else
    assert(e_inv > 0, [emsg ' ; e_inv<=0']);
end

== matlab function sampleModel7424_pp_1_1/emi_209 ==
  data: o input; e input
function  fcn(o, e)
o_inv = o^-1;
e_inv = e^-1;

emsg = 'sampleModel7424_pp_1_1/emi_209';
 
if(o == e)
    assert(o_inv == e_inv, [emsg ' ; o_inv~=e_inv']);
    return;
end
 
if(o_inv > 0)
    assert(e_inv < 0, [emsg ' ; e_inv>=0']);
else
    assert(e_inv > 0, [emsg ' ; e_inv<=0']);
end

== matlab function sampleModel7424_pp_1_1/cfblk148/cfblk19/emi_211 ==
  data: o input; e input
function  fcn(o, e)
o_inv = o^-1;
e_inv = e^-1;

emsg = 'sampleModel7424_pp_1_1/cfblk148/cfblk19/emi_211';
 
if(o == e)
    assert(o_inv == e_inv, [emsg ' ; o_inv~=e_inv']);
    return;
end
 
if(o_inv > 0)
    assert(e_inv < 0, [emsg ' ; e_inv>=0']);
else
    assert(e_inv > 0, [emsg ' ; e_inv<=0']);
end

== matlab function sampleModel7424_pp_1_1/cfblk142/cfblk19/emi_213 ==
  data: o input; e input
function  fcn(o, e)
o_inv = o^-1;
e_inv = e^-1;

emsg = 'sampleModel7424_pp_1_1/cfblk142/cfblk19/emi_213';
 
if(o == e)
    assert(o_inv == e_inv, [emsg ' ; o_inv~=e_inv']);
    return;
end
 
if(o_inv > 0)
    assert(e_inv < 0, [emsg ' ; e_inv>=0']);
else
    assert(e_inv > 0, [emsg ' ; e_inv<=0']);
end

== matlab function sampleModel7424_pp_1_1/cfblk148/emi_215 ==
  data: o input; e input
function  fcn(o, e)
o_inv = o^-1;
e_inv = e^-1;

emsg = 'sampleModel7424_pp_1_1/cfblk148/emi_215';
 
if(o == e)
    assert(o_inv == e_inv, [emsg ' ; o_inv~=e_inv']);
    return;
end
 
if(o_inv > 0)
    assert(e_inv < 0, [emsg ' ; e_inv>=0']);
else
    assert(e_inv > 0, [emsg ' ; e_inv<=0']);
end

== matlab function sampleModel7424_pp_1_1/cfblk141/emi_217 ==
  data: o input; e input
function  fcn(o, e)
o_inv = o^-1;
e_inv = e^-1;

emsg = 'sampleModel7424_pp_1_1/cfblk141/emi_217';
 
if(o == e)
    assert(o_inv == e_inv, [emsg ' ; o_inv~=e_inv']);
    return;
end
 
if(o_inv > 0)
    assert(e_inv < 0, [emsg ' ; e_inv>=0']);
else
    assert(e_inv > 0, [emsg ' ; e_inv<=0']);
end

== matlab function sampleModel7424_pp_1_1/cfblk126/cfblk13/emi_219 ==
  data: o input; e input
function  fcn(o, e)
o_inv = o^-1;
e_inv = e^-1;

emsg = 'sampleModel7424_pp_1_1/cfblk126/cfblk13/emi_219';
 
if(o == e)
    assert(o_inv == e_inv, [emsg ' ; o_inv~=e_inv']);
    return;
end
 
if(o_inv > 0)
    assert(e_inv < 0, [emsg ' ; e_inv>=0']);
else
    assert(e_inv > 0, [emsg ' ; e_inv<=0']);
end

== matlab function sampleModel7424_pp_1_1/cfblk124/cfblk15/emi_221 ==
  data: o input; e input
function  fcn(o, e)
o_inv = o^-1;
e_inv = e^-1;

emsg = 'sampleModel7424_pp_1_1/cfblk124/cfblk15/emi_221';
 
if(o == e)
    assert(o_inv == e_inv, [emsg ' ; o_inv~=e_inv']);
    return;
end
 
if(o_inv > 0)
    assert(e_inv < 0, [emsg ' ; e_inv>=0']);
else
    assert(e_inv > 0, [emsg ' ; e_inv<=0']);
end

== matlab function sampleModel7424_pp_1_1/emi_223 ==
  data: o input; e input
function  fcn(o, e)
o_inv = o^-1;
e_inv = e^-1;

emsg = 'sampleModel7424_pp_1_1/emi_223';
 
if(o == e)
    assert(o_inv == e_inv, [emsg ' ; o_inv~=e_inv']);
    return;
end
 
if(o_inv > 0)
    assert(e_inv < 0, [emsg ' ; e_inv>=0']);
else
    assert(e_inv > 0, [emsg ' ; e_inv<=0']);
end

== matlab function sampleModel7424_pp_1_1/cfblk142/emi_225 ==
  data: o input; e input
function  fcn(o, e)
o_inv = o^-1;
e_inv = e^-1;

emsg = 'sampleModel7424_pp_1_1/cfblk142/emi_225';
 
if(o == e)
    assert(o_inv == e_inv, [emsg ' ; o_inv~=e_inv']);
    return;
end
 
if(o_inv > 0)
    assert(e_inv < 0, [emsg ' ; e_inv>=0']);
else
    assert(e_inv > 0, [emsg ' ; e_inv<=0']);
end

== matlab function sampleModel7424_pp_1_1/cfblk136/emi_227 ==
  data: o input; e input
function  fcn(o, e)
o_inv = o^-1;
e_inv = e^-1;

emsg = 'sampleModel7424_pp_1_1/cfblk136/emi_227';
 
if(o == e)
    assert(o_inv == e_inv, [emsg ' ; o_inv~=e_inv']);
    return;
end
 
if(o_inv > 0)
    assert(e_inv < 0, [emsg ' ; e_inv>=0']);
else
    assert(e_inv > 0, [emsg ' ; e_inv<=0']);
end

== matlab function sampleModel7424_pp_1_1/cfblk142/emi_229 ==
  data: o input; e input
function  fcn(o, e)
o_inv = o^-1;
e_inv = e^-1;

emsg = 'sampleModel7424_pp_1_1/cfblk142/emi_229';
 
if(o == e)
    assert(o_inv == e_inv, [emsg ' ; o_inv~=e_inv']);
    return;
end
 
if(o_inv > 0)
    assert(e_inv < 0, [emsg ' ; e_inv>=0']);
else
    assert(e_inv > 0, [emsg ' ; e_inv<=0']);
end

== matlab function sampleModel7424_pp_1_1/cfblk125/cfblk12/emi_231 ==
  data: o input; e input
function  fcn(o, e)
o_inv = o^-1;
e_inv = e^-1;

emsg = 'sampleModel7424_pp_1_1/cfblk125/cfblk12/emi_231';
 
if(o == e)
    assert(o_inv == e_inv, [emsg ' ; o_inv~=e_inv']);
    return;
end
 
if(o_inv > 0)
    assert(e_inv < 0, [emsg ' ; e_inv>=0']);
else
    assert(e_inv > 0, [emsg ' ; e_inv<=0']);
end

== matlab function sampleModel7424_pp_1_1/cfblk133/emi_233 ==
  data: o input; e input
function  fcn(o, e)
o_inv = o^-1;
e_inv = e^-1;

emsg = 'sampleModel7424_pp_1_1/cfblk133/emi_233';
 
if(o == e)
    assert(o_inv == e_inv, [emsg ' ; o_inv~=e_inv']);
    return;
end
 
if(o_inv > 0)
    assert(e_inv < 0, [emsg ' ; e_inv>=0']);
else
    assert(e_inv > 0, [emsg ' ; e_inv<=0']);
end

== matlab function sampleModel7424_pp_1_1/emi_235 ==
  data: o input; e input
function  fcn(o, e)
o_inv = o^-1;
e_inv = e^-1;

emsg = 'sampleModel7424_pp_1_1/emi_235';
 
if(o == e)
    assert(o_inv == e_inv, [emsg ' ; o_inv~=e_inv']);
    return;
end
 
if(o_inv > 0)
    assert(e_inv < 0, [emsg ' ; e_inv>=0']);
else
    assert(e_inv > 0, [emsg ' ; e_inv<=0']);
end

== matlab function sampleModel7424_pp_1_1/cfblk124/emi_237 ==
  data: o input; e input
function  fcn(o, e)
o_inv = o^-1;
e_inv = e^-1;

emsg = 'sampleModel7424_pp_1_1/cfblk124/emi_237';
 
if(o == e)
    assert(o_inv == e_inv, [emsg ' ; o_inv~=e_inv']);
    return;
end
 
if(o_inv > 0)
    assert(e_inv < 0, [emsg ' ; e_inv>=0']);
else
    assert(e_inv > 0, [emsg ' ; e_inv<=0']);
end

== matlab function sampleModel7424_pp_1_1/cfblk125/cfblk12/emi_239 ==
  data: o input; e input
function  fcn(o, e)
o_inv = o^-1;
e_inv = e^-1;

emsg = 'sampleModel7424_pp_1_1/cfblk125/cfblk12/emi_239';
 
if(o == e)
    assert(o_inv == e_inv, [emsg ' ; o_inv~=e_inv']);
    return;
end
 
if(o_inv > 0)
    assert(e_inv < 0, [emsg ' ; e_inv>=0']);
else
    assert(e_inv > 0, [emsg ' ; e_inv<=0']);
end

== matlab function sampleModel7424_pp_1_1/cfblk126/emi_241 ==
  data: o input; e input
function  fcn(o, e)
o_inv = o^-1;
e_inv = e^-1;

emsg = 'sampleModel7424_pp_1_1/cfblk126/emi_241';
 
if(o == e)
    assert(o_inv == e_inv, [emsg ' ; o_inv~=e_inv']);
    return;
end
 
if(o_inv > 0)
    assert(e_inv < 0, [emsg ' ; e_inv>=0']);
else
    assert(e_inv > 0, [emsg ' ; e_inv<=0']);
end

== matlab function sampleModel7424_pp_1_1/cfblk141/emi_243 ==
  data: o input; e input
function  fcn(o, e)
o_inv = o^-1;
e_inv = e^-1;

emsg = 'sampleModel7424_pp_1_1/cfblk141/emi_243';
 
if(o == e)
    assert(o_inv == e_inv, [emsg ' ; o_inv~=e_inv']);
    return;
end
 
if(o_inv > 0)
    assert(e_inv < 0, [emsg ' ; e_inv>=0']);
else
    assert(e_inv > 0, [emsg ' ; e_inv<=0']);
end

== matlab function sampleModel7424_pp_1_1/cfblk138/emi_245 ==
  data: o input; e input
function  fcn(o, e)
o_inv = o^-1;
e_inv = e^-1;

emsg = 'sampleModel7424_pp_1_1/cfblk138/emi_245';
 
if(o == e)
    assert(o_inv == e_inv, [emsg ' ; o_inv~=e_inv']);
    return;
end
 
if(o_inv > 0)
    assert(e_inv < 0, [emsg ' ; e_inv>=0']);
else
    assert(e_inv > 0, [emsg ' ; e_inv<=0']);
end

== matlab function sampleModel7424_pp_1_1/emi_247 ==
  data: o input; e input
function  fcn(o, e)
o_inv = o^-1;
e_inv = e^-1;

emsg = 'sampleModel7424_pp_1_1/emi_247';
 
if(o == e)
    assert(o_inv == e_inv, [emsg ' ; o_inv~=e_inv']);
    return;
end
 
if(o_inv > 0)
    assert(e_inv < 0, [emsg ' ; e_inv>=0']);
else
    assert(e_inv > 0, [emsg ' ; e_inv<=0']);
end

== matlab function sampleModel7424_pp_1_1/emi_249 ==
  data: o input; e input
function  fcn(o, e)
o_inv = o^-1;
e_inv = e^-1;

emsg = 'sampleModel7424_pp_1_1/emi_249';
 
if(o == e)
    assert(o_inv == e_inv, [emsg ' ; o_inv~=e_inv']);
    return;
end
 
if(o_inv > 0)
    assert(e_inv < 0, [emsg ' ; e_inv>=0']);
else
    assert(e_inv > 0, [emsg ' ; e_inv<=0']);
end

== matlab function sampleModel7424_pp_1_1/cfblk133/emi_251 ==
  data: o input; e input
function  fcn(o, e)
o_inv = o^-1;
e_inv = e^-1;

emsg = 'sampleModel7424_pp_1_1/cfblk133/emi_251';
 
if(o == e)
    assert(o_inv == e_inv, [emsg ' ; o_inv~=e_inv']);
    return;
end
 
if(o_inv > 0)
    assert(e_inv < 0, [emsg ' ; e_inv>=0']);
else
    assert(e_inv > 0, [emsg ' ; e_inv<=0']);
end

== matlab function sampleModel7424_pp_1_1/emi_253 ==
  data: o input; e input
function  fcn(o, e)
o_inv = o^-1;
e_inv = e^-1;

emsg = 'sampleModel7424_pp_1_1/emi_253';
 
if(o == e)
    assert(o_inv == e_inv, [emsg ' ; o_inv~=e_inv']);
    return;
end
 
if(o_inv > 0)
    assert(e_inv < 0, [emsg ' ; e_inv>=0']);
else
    assert(e_inv > 0, [emsg ' ; e_inv<=0']);
end

== matlab function sampleModel7424_pp_1_1/cfblk124/cfblk15/emi_255 ==
  data: o input; e input
function  fcn(o, e)
o_inv = o^-1;
e_inv = e^-1;

emsg = 'sampleModel7424_pp_1_1/cfblk124/cfblk15/emi_255';
 
if(o == e)
    assert(o_inv == e_inv, [emsg ' ; o_inv~=e_inv']);
    return;
end
 
if(o_inv > 0)
    assert(e_inv < 0, [emsg ' ; e_inv>=0']);
else
    assert(e_inv > 0, [emsg ' ; e_inv<=0']);
end

== matlab function sampleModel7424_pp_1_1/cfblk148/emi_257 ==
  data: o input; e input
function  fcn(o, e)
o_inv = o^-1;
e_inv = e^-1;

emsg = 'sampleModel7424_pp_1_1/cfblk148/emi_257';
 
if(o == e)
    assert(o_inv == e_inv, [emsg ' ; o_inv~=e_inv']);
    return;
end
 
if(o_inv > 0)
    assert(e_inv < 0, [emsg ' ; e_inv>=0']);
else
    assert(e_inv > 0, [emsg ' ; e_inv<=0']);
end

== matlab function sampleModel7424_pp_1_1/cfblk126/emi_259 ==
  data: o input; e input
function  fcn(o, e)
o_inv = o^-1;
e_inv = e^-1;

emsg = 'sampleModel7424_pp_1_1/cfblk126/emi_259';
 
if(o == e)
    assert(o_inv == e_inv, [emsg ' ; o_inv~=e_inv']);
    return;
end
 
if(o_inv > 0)
    assert(e_inv < 0, [emsg ' ; e_inv>=0']);
else
    assert(e_inv > 0, [emsg ' ; e_inv<=0']);
end

== matlab function sampleModel7424_pp_1_1/cfblk134/emi_261 ==
  data: o input; e input
function  fcn(o, e)
o_inv = o^-1;
e_inv = e^-1;

emsg = 'sampleModel7424_pp_1_1/cfblk134/emi_261';
 
if(o == e)
    assert(o_inv == e_inv, [emsg ' ; o_inv~=e_inv']);
    return;
end
 
if(o_inv > 0)
    assert(e_inv < 0, [emsg ' ; e_inv>=0']);
else
    assert(e_inv > 0, [emsg ' ; e_inv<=0']);
end

== matlab function sampleModel7424_pp_1_1/cfblk141/emi_263 ==
  data: o input; e input
function  fcn(o, e)
o_inv = o^-1;
e_inv = e^-1;

emsg = 'sampleModel7424_pp_1_1/cfblk141/emi_263';
 
if(o == e)
    assert(o_inv == e_inv, [emsg ' ; o_inv~=e_inv']);
    return;
end
 
if(o_inv > 0)
    assert(e_inv < 0, [emsg ' ; e_inv>=0']);
else
    assert(e_inv > 0, [emsg ' ; e_inv<=0']);
end

== matlab function sampleModel7424_pp_1_1/cfblk126/cfblk15/emi_265 ==
  data: o input; e input
function  fcn(o, e)
o_inv = o^-1;
e_inv = e^-1;

emsg = 'sampleModel7424_pp_1_1/cfblk126/cfblk15/emi_265';
 
if(o == e)
    assert(o_inv == e_inv, [emsg ' ; o_inv~=e_inv']);
    return;
end
 
if(o_inv > 0)
    assert(e_inv < 0, [emsg ' ; e_inv>=0']);
else
    assert(e_inv > 0, [emsg ' ; e_inv<=0']);
end
